simulink model "fileSimulinl"  (R2014a)
settings: Solver=ode45  StartTime=0.0  StopTime=10  RelTol=1e-3
libraries: cstblocks x3, simulink x1
settings Model: Creator=User  LastModifiedBy=User

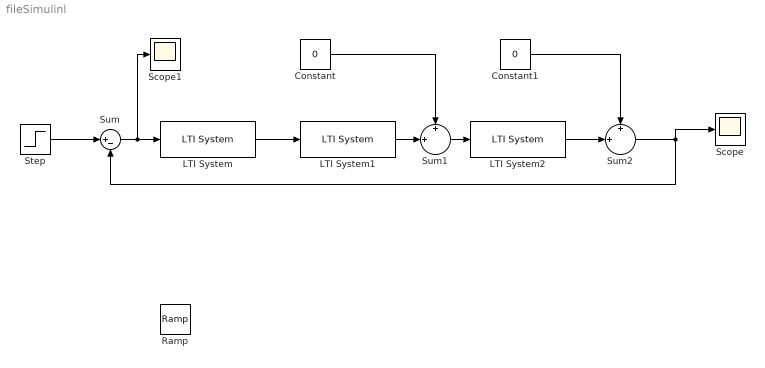
== system fileSimulinl ==
  Constant : Constant  Value=0
  Constant1 : Constant  Value=0
  LTI System : cstblocks/LTI System  sys=Cz3  IC=[]
  LTI System1 : cstblocks/LTI System  sys=F1  IC=[]
  LTI System2 : cstblocks/LTI System  sys=F2  IC=[]
  Ramp : simulink/Sources/Ramp  slope=1  start=0  X0=0
  Scope : Scope
  Scope1 : Scope
  Step : Step  Time=0  SampleTime=0
  Sum : Sum  Inputs=|+-
  Sum1 : Sum  Inputs=+|+||
  Sum2 : Sum  Inputs=+|+||
  wires:
  Sum/1 -> Scope1/1, LTI System/1
  LTI System/1 -> LTI System1/1
  Constant/1 -> Sum1/1
  LTI System1/1 -> Sum1/2
  Sum1/1 -> LTI System2/1
  LTI System2/1 -> Sum2/2
  Constant1/1 -> Sum2/1
  Sum2/1 -> Scope/1, Sum/2
  Step/1 -> Sum/1
